simulink model "cstr"  (Simulink 8.8)
settings: Solver=ode45  StartTime=0.0  StopTime=1000.0  RelTol=1e-3  EnableMultiTasking=on
settings Model: Creator=The MathWorks, Inc.  LastModifiedBy=The MathWorks, Inc.  ExtModeTrigMode=oneshot  ExtModeArmWhenConnect=off
settings DataIOCC: LimitDataPoints=off  SignalLoggingSaveFormat=Dataset
settings OptimizationCC: BlockReduction=off  BooleanDataType=off  InitFltsAndDblsToZero=on
settings DebuggingCC: SaveWithParameterizedLinksMsg=none  SignalResolutionControl=TryResolveAllWithWarning  MultiTaskDSMMsg=warning  MultiTaskCondExecSysMsg=none  StateNameClashWarn=none  StrictBusMsg=None
settings HardwareCC: TargetUnknown=on
settings GRTTargetCC: TargetFcnLib=ansi_tfl_tmw.mat  GeneratePreprocessorConditionals=Use local settings

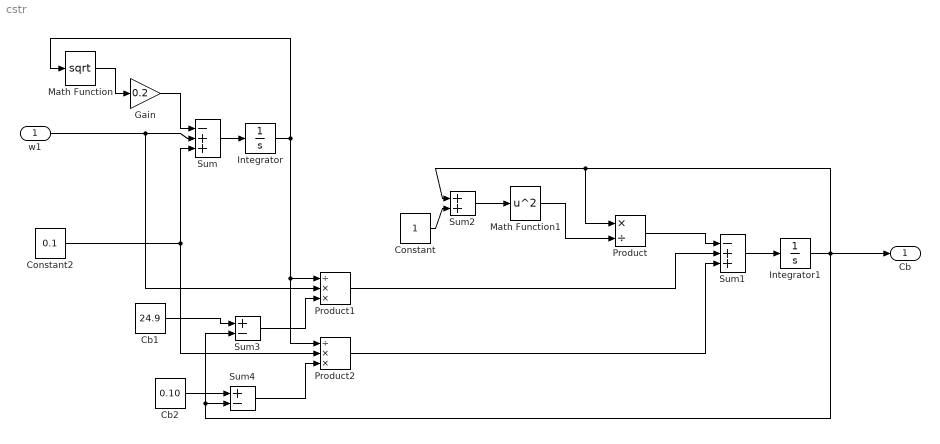
== system cstr ==
  w1 : Inport
  Cb1 : Constant  Value=24.9
  Cb2 : Constant  Value=0.10
  Constant : Constant
  Constant2 : Constant  Value=0.1
  Gain : Gain  Gain=0.2  SaturateOnIntegerOverflow=on  OutDataTypeStr=Inherit: Same as input  ParamDataTypeStr=Inherit: Same as input
  Integrator : Integrator  InitialCondition=30  LimitOutput=on  LowerSaturationLimit=1
  Integrator1 : Integrator  InitialCondition=22
  Math Function : Math  Operator=sqrt  SaturateOnIntegerOverflow=on
  Math Function1 : Math  Operator=square  SaturateOnIntegerOverflow=on
  Product : Product  Inputs=*/  SaturateOnIntegerOverflow=on  RndMeth=Zero  InputSameDT=on  OutDataTypeStr=Inherit: Same as first input
  Product1 : Product  Inputs=/**  SaturateOnIntegerOverflow=on  RndMeth=Zero  InputSameDT=on  OutDataTypeStr=Inherit: Same as first input
  Product2 : Product  Inputs=/**  SaturateOnIntegerOverflow=on  RndMeth=Zero  InputSameDT=on  OutDataTypeStr=Inherit: Same as first input
  Sum : Sum  Inputs=-++  SaturateOnIntegerOverflow=on  InputSameDT=on  OutDataTypeStr=Inherit: Same as first input
  Sum1 : Sum  Inputs=-++  SaturateOnIntegerOverflow=on  InputSameDT=on  OutDataTypeStr=Inherit: Same as first input
  Sum2 : Sum  SaturateOnIntegerOverflow=on  InputSameDT=on  OutDataTypeStr=Inherit: Same as first input
  Sum3 : Sum  Inputs=+-  SaturateOnIntegerOverflow=on  InputSameDT=on  OutDataTypeStr=Inherit: Same as first input
  Sum4 : Sum  Inputs=+-  SaturateOnIntegerOverflow=on  InputSameDT=on  OutDataTypeStr=Inherit: Same as first input
  Cb : Outport
  wires:
  Sum/1 -> Integrator/1
  Gain/1 -> Sum/1
  Math Function/1 -> Gain/1
  Integrator/1 -> Math Function/1, Product1/1, Product2/1
  Cb1/1 -> Sum3/1
  Cb2/1 -> Sum4/1
  Sum3/1 -> Product1/3
  Sum4/1 -> Product2/3
  Constant/1 -> Sum2/2
  Sum2/1 -> Math Function1/1
  Sum1/1 -> Integrator1/1
  Math Function1/1 -> Product/2
  Product/1 -> Sum1/1
  Product1/1 -> Sum1/2
  Product2/1 -> Sum1/3
  w1/1 -> Sum/2, Product1/2
  Constant2/1 -> Sum/3, Product2/2
  Integrator1/1 -> Sum3/2, Sum4/2, Sum2/1, Product/1, Cb/1
